simulink model "homework1"  (R2023b)
settings: Solver=VariableStepAuto  StartTime=0.0  StopTime=10.0  RelTol=1e-3
values from neighbouring files (symbols this model uses):
  Aprime = T^(-1)*A*T    [homework1.m]
  Bprime = T^(-1)*B    [homework1.m]
  denp = [3 1]    [homework1.m]
  h = 6.5    [homework1.m]
  I = eye(size(A))    [homework1.m]
  K = 6*(-A)    [homework1.m]    (also in script_radmila.m = 1.2)
  kr = (Cprime*((Bprime*K-Aprime)^(-1))*Bprime)^(-1)    [homework1.m]
  nump = [0 2]    [homework1.m]
  s = tf('s')    [homework1.m]
libraries: cstblocks x17
settings Model: Creator=klysm  LastModifiedBy=klysm

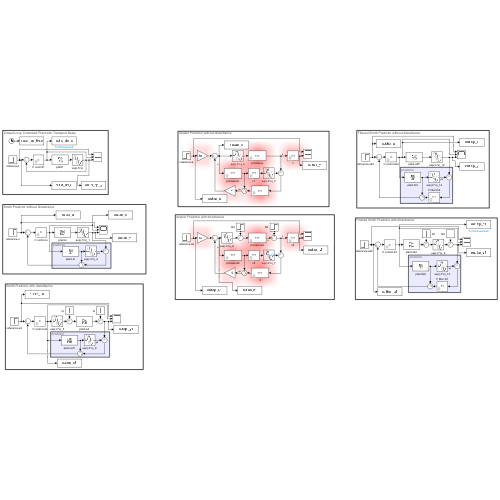
[thumbnail: Simulink's stored preview of the top-level diagram]
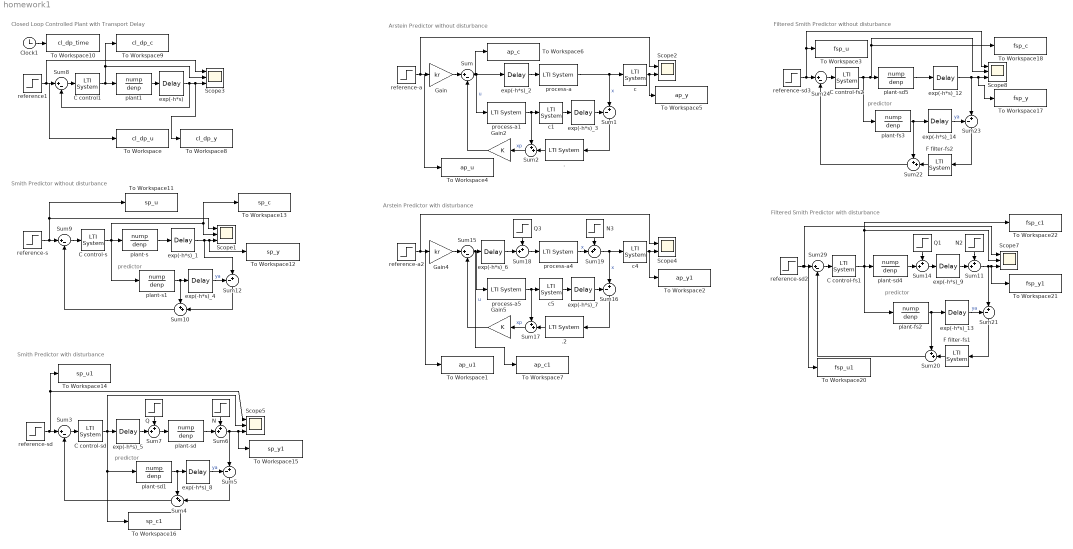
== system homework1 ==
  note: Arstein Predictor with disturbance
  note: Arstein Predictor without disturbance
  note: Smith Predictor without disturbance
  note: Closed Loop Controlled Plant with Transport Delay
  note: predictor
  note: predictor
  note: Smith Predictor with disturbance
  note: predictor
  note: Filtered Smith Predictor with disturbance
  note: predictor
  note: Filtered Smith Predictor without disturbance
  . : cstblocks/LTI System  sys=exp(Aprime*h)  IC=[]  PadeOrder=0
  .2 : cstblocks/LTI System  sys=exp(Aprime*h)  IC=[]  PadeOrder=0
  C control-fs1 : cstblocks/LTI System  sys=C  IC=[]  PadeOrder=0
  C control-fs2 : cstblocks/LTI System  sys=C  IC=[]  PadeOrder=0
  C control-s : cstblocks/LTI System  sys=C  IC=[]  PadeOrder=0
  C control-sd : cstblocks/LTI System  sys=C  IC=[]  PadeOrder=0
  C control1 : cstblocks/LTI System  sys=C  IC=[]  PadeOrder=0
  Clock1 : Clock
  F filter-fs1 : cstblocks/LTI System  sys=F1  IC=[]  PadeOrder=0
  F filter-fs2 : cstblocks/LTI System  sys=F1  IC=[]  PadeOrder=0
  Gain : Gain  Gain=kr
  Gain2 : Gain  Gain=K
  Gain4 : Gain  Gain=kr
  Gain5 : Gain  Gain=K
  N : Step  Time=20  After=0.2  SampleTime=0
  N2 : Step  Time=20  After=0.2  SampleTime=0
  N3 : Step  Time=20  After=0.2  SampleTime=0
  Q : Step  Time=10  After=0.2  SampleTime=0
  Q1 : Step  Time=10  After=0.2  SampleTime=0
  Q3 : Step  Time=10  After=0.2  SampleTime=0
  Scope{1,3,5,7..8} (5 alike) : Scope  NumInputPorts=3
  Scope2 : Scope  NumInputPorts=2
  Scope4 : Scope  NumInputPorts=2
  Sum{,3,8..9,15,24,29} (7 alike) : Sum  Inputs=|+-
  Sum{1,5,12,16,21,23} (6 alike) : Sum  Inputs=-+|
  Sum{2,4,6..7,10..11,14,17..20,22} (12 alike) : Sum  Inputs=++|
  To Workspace : ToWorkspace  VariableName=cl_dp_u  SampleTime=-1
  To Workspace1 : ToWorkspace  VariableName=ap_u1  SampleTime=-1
  To Workspace10 : ToWorkspace  VariableName=cl_dp_time  SampleTime=-1
  To Workspace11 : ToWorkspace  VariableName=sp_u  SampleTime=-1
  To Workspace12 : ToWorkspace  VariableName=sp_y  SampleTime=-1
  To Workspace13 : ToWorkspace  VariableName=sp_c  SampleTime=-1
  To Workspace14 : ToWorkspace  VariableName=sp_u1  SampleTime=-1
  To Workspace15 : ToWorkspace  VariableName=sp_y1  SampleTime=-1
  To Workspace16 : ToWorkspace  VariableName=sp_c1  SampleTime=-1
  To Workspace17 : ToWorkspace  VariableName=fsp_y  SampleTime=-1
  To Workspace18 : ToWorkspace  VariableName=fsp_c  SampleTime=-1
  To Workspace2 : ToWorkspace  VariableName=ap_y1  SampleTime=-1
  To Workspace20 : ToWorkspace  VariableName=fsp_u1  SampleTime=-1
  To Workspace21 : ToWorkspace  VariableName=fsp_y1  SampleTime=-1
  To Workspace22 : ToWorkspace  VariableName=fsp_c1  SampleTime=-1
  To Workspace3 : ToWorkspace  VariableName=fsp_u  SampleTime=-1
  To Workspace4 : ToWorkspace  VariableName=ap_u  SampleTime=-1
  To Workspace5 : ToWorkspace  VariableName=ap_y  SampleTime=-1
  To Workspace6 : ToWorkspace  VariableName=ap_c  SampleTime=-1
  To Workspace7 : ToWorkspace  VariableName=ap_c1  SampleTime=-1
  To Workspace8 : ToWorkspace  VariableName=cl_dp_y  SampleTime=-1
  To Workspace9 : ToWorkspace  VariableName=cl_dp_c  SampleTime=-1
  c{,1,4..5} (4 alike) : cstblocks/LTI System  sys=Cprime  IC=[]  PadeOrder=0
  exp(-h*s) : TransportDelay
  exp(-h*s)_{1..9,12..14} (12 alike) : TransportDelay  DelayTime=h
  plant-fs2 : TransferFcn  Numerator=nump  Denominator=denp
  plant-fs3 : TransferFcn  Numerator=nump  Denominator=denp
  plant-s : TransferFcn  Numerator=nump  Denominator=denp
  plant-s1 : TransferFcn  Numerator=nump  Denominator=denp
  plant-sd{,1,4..5} (4 alike) : TransferFcn  Numerator=nump  Denominator=denp
  plant1 : TransferFcn  Numerator=nump  Denominator=denp
  process-a{,1,4..5} (4 alike) : cstblocks/LTI System  sys=inv(s*I-Aprime)*Bprime  IC=[]  PadeOrder=0
  reference-a : Step  Time=0  SampleTime=0
  reference-a2 : Step  Time=0  SampleTime=0
  reference-s : Step  Time=0  SampleTime=0
  reference-sd : Step  Time=0  SampleTime=0
  reference-sd2 : Step  Time=0  SampleTime=0
  reference-sd3 : Step  Time=0  SampleTime=0
  reference1 : Step  Time=0  SampleTime=0
  wires:
  Q3/1 -> Sum18/1
  exp(-h*s)_7/1 -> Sum16/1
  Sum15/1 -> process-a5/1, exp(-h*s)_6/1, To Workspace7/1  "u"
  Sum19/1 -> c4/1, Sum16/2  "x"
  process-a5/1 -> c5/1, Sum17/1
  reference-a2/1 -> To Workspace1/1, Scope4/1, Gain4/1
  Sum17/1 -> Gain5/1  "xp"
  c5/1 -> exp(-h*s)_7/1
  Sum2/1 -> Gain2/1  "xp"
  c4/1 -> To Workspace2/1, Scope4/2
  .2/1 -> Sum17/2
  Sum18/1 -> process-a4/1
  Gain4/1 -> Sum15/1
  N3/1 -> Sum19/1
  exp(-h*s)_2/1 -> process-a/1
  c1/1 -> exp(-h*s)_3/1
  exp(-h*s)_3/1 -> Sum1/1
  Gain5/1 -> Sum15/2
  ./1 -> Sum2/2
  Gain2/1 -> Sum/2
  Sum16/1 -> .2/1
  process-a/1 -> c/1, Sum1/2  "x"
  Sum1/1 -> ./1
  c/1 -> To Workspace5/1, Scope2/2
  process-a1/1 -> c1/1, Sum2/1
  Gain/1 -> Sum/1
  Sum/1 -> exp(-h*s)_2/1, process-a1/1, To Workspace6/1  "u"
  process-a4/1 -> Sum19/2  "x"
  reference-a/1 -> To Workspace4/1, Scope2/1, Gain/1
  exp(-h*s)_6/1 -> Sum18/2
  plant-sd/1 -> Sum6/2
  plant-s/1 -> exp(-h*s)_1/1
  plant-s1/1 -> Sum10/1, exp(-h*s)_4/1
  Sum6/1 -> To Workspace15/1, Scope5/3, Sum5/2
  Sum7/1 -> plant-sd/1
  Q/1 -> Sum7/1
  Sum4/1 -> Sum3/2
  Sum9/1 -> C control-s/1
  exp(-h*s)_5/1 -> Sum7/2
  Sum10/1 -> Sum9/2
  exp(-h*s)_4/1 -> Sum12/1  "ya"
  reference-s/1 -> To Workspace11/1, Scope1/1, Sum9/1
  plant1/1 -> exp(-h*s)/1
  C control-sd/1 -> To Workspace16/1, plant-sd1/1, exp(-h*s)_5/1, Scope5/2
  reference-sd/1 -> To Workspace14/1, Scope5/1, Sum3/1
  exp(-h*s)_8/1 -> Sum5/1  "ya"
  Sum12/1 -> Sum10/2
  exp(-h*s)_1/1 -> Sum12/2, To Workspace12/1, Scope1/3
  Clock1/1 -> To Workspace10/1
  Sum3/1 -> C control-sd/1
  exp(-h*s)/1 -> To Workspace8/1, Scope3/3, Sum8/2
  Sum8/1 -> C control1/1
  N/1 -> Sum6/1
  C control-s/1 -> To Workspace13/1, Scope1/2, plant-s/1, plant-s1/1
  C control1/1 -> To Workspace9/1, Scope3/2, plant1/1
  plant-sd1/1 -> Sum4/1, exp(-h*s)_8/1
  Sum5/1 -> Sum4/2
  reference1/1 -> To Workspace/1, Sum8/1, Scope3/1
  Sum14/1 -> exp(-h*s)_9/1
  C control-fs2/1 -> plant-sd5/1, Scope8/2, To Workspace18/1, plant-fs3/1
  plant-sd4/1 -> Sum14/2
  exp(-h*s)_14/1 -> Sum23/1  "ya"
  F filter-fs1/1 -> Sum20/2
  reference-sd3/1 -> To Workspace3/1, Scope8/1, Sum24/1
  Sum22/1 -> Sum24/2
  Sum21/1 -> F filter-fs1/1
  exp(-h*s)_12/1 -> To Workspace17/1, Scope8/3, Sum23/2
  F filter-fs2/1 -> Sum22/2
  C control-fs1/1 -> To Workspace22/1, Scope7/2, plant-fs2/1, plant-sd4/1
  plant-sd5/1 -> exp(-h*s)_12/1
  Sum23/1 -> F filter-fs2/1
  Sum24/1 -> C control-fs2/1
  N2/1 -> Sum11/1
  reference-sd2/1 -> To Workspace20/1, Scope7/1, Sum29/1
  Sum29/1 -> C control-fs1/1
  Sum11/1 -> To Workspace21/1, Scope7/3, Sum21/2
  plant-fs2/1 -> exp(-h*s)_13/1, Sum20/1
  exp(-h*s)_9/1 -> Sum11/2
  exp(-h*s)_13/1 -> Sum21/1  "ya"
  Sum20/1 -> Sum29/2
  Q1/1 -> Sum14/1
  plant-fs3/1 -> exp(-h*s)_14/1, Sum22/1
